simulink model "Machine_Learning"  (R2021b)
settings: Solver=FixedStepAuto  StartTime=0.0  StopTime=1.3  FixedStep=Ts  RelTol=1e-3
model workspace (MAT data in the model file):
  Motor_Gain = 1
values from neighbouring files (symbols this model uses):
  Gain = x(i)    [LS_simulation.m]
  J = 7.65e-3    (= 0.00765)    [Hyperparamter_Optimization.m]    (also in LS_simulation.m)
  Ka = 6.4898    [Hyperparamter_Optimization.m]    (also in LS_simulation.m)
  Kt = 0.4769    [Hyperparamter_Optimization.m]    (also in LS_simulation.m)
  rg = 1.5915    [LS_simulation.m]
settings Model: Creator=user  LastModifiedBy=Duncan
settings SolverCC: AlgebraicLoopSolver=TrustRegion
settings DebuggingCC: SFMachineParentedDataDiag=warning

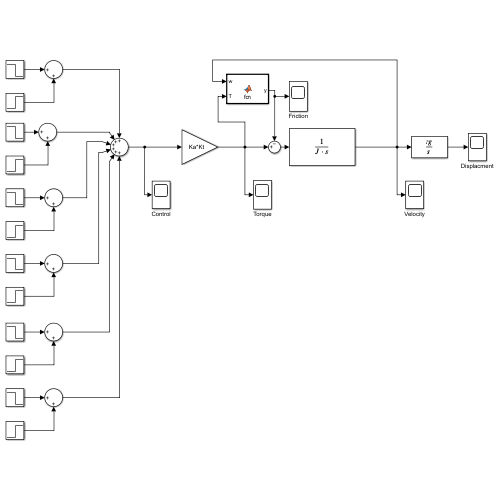
[thumbnail: Simulink's stored preview of the top-level diagram]
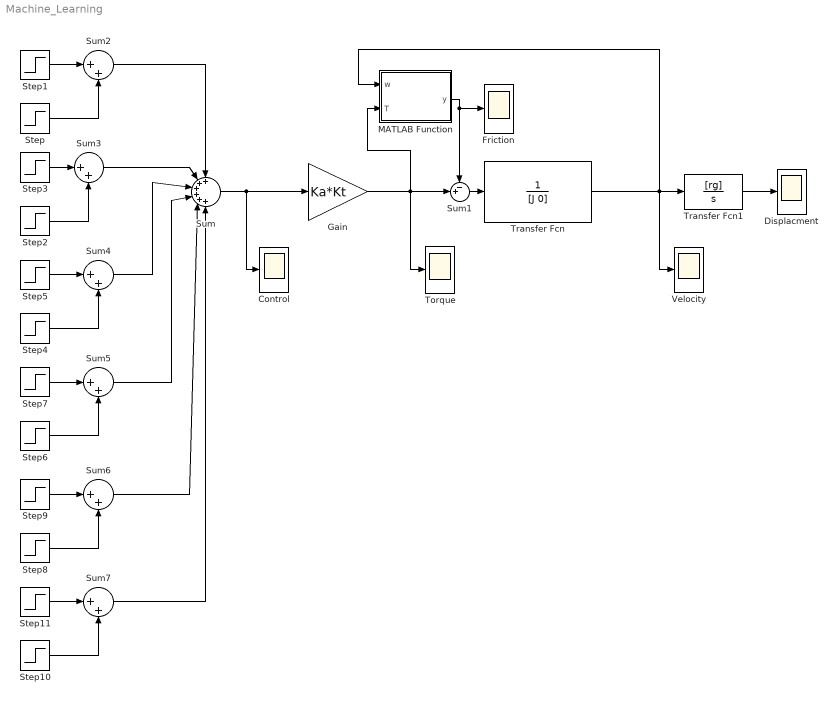
== system Machine_Learning ==
  Control : Scope
  Displacment : Scope
  Friction : Scope
  Gain : Gain  Gain=Ka*Kt
  MATLAB Function : MATLAB Function  TreatAsAtomicUnit=on
  Step : Step  Time=0.2  After=0.2*Gain  SampleTime=0
  Step1 : Step  Time=0.1  After=-0.1*Gain  SampleTime=0
  Step10 : Step  Time=1.2  After=0.1*Gain  SampleTime=0
  Step11 : Step  Time=1.1  After=-0.2*Gain  SampleTime=0
  Step2 : Step  Time=0.4  After=0.4*Gain  SampleTime=0
  Step3 : Step  Time=0.3  After=-0.3*Gain  SampleTime=0
  Step4 : Step  Time=0.6  After=0.6*Gain  SampleTime=0
  Step5 : Step  Time=0.5  After=-0.5*Gain  SampleTime=0
  Step6 : Step  Time=0.8  After=0.5*Gain  SampleTime=0
  Step7 : Step  Time=0.7  After=-0.6*Gain  SampleTime=0
  Step8 : Step  After=0.3*Gain  SampleTime=0
  Step9 : Step  Time=0.9  After=-0.4*Gain  SampleTime=0
  Sum : Sum  Inputs=++++++
  Sum1 : Sum  Inputs=-+|
  Sum{2..7} (6 alike) : Sum  Inputs=|++
  Torque : Scope
  Transfer Fcn : TransferFcn  Denominator=[J 0]
  Transfer Fcn1 : TransferFcn  Numerator=[rg]  Denominator=[1 0]
  Velocity : Scope
  wires:
  Gain/1 -> MATLAB Function/2(T), Sum1/2, Torque/1
  Sum1/1 -> Transfer Fcn/1
  MATLAB Function/1(y) -> Friction/1, Sum1/1
  Transfer Fcn1/1 -> Displacment/1
  Step1/1 -> Sum2/1
  Sum2/1 -> Sum/1
  Sum3/1 -> Sum/2
  Sum4/1 -> Sum/3
  Sum5/1 -> Sum/4
  Sum6/1 -> Sum/5
  Sum7/1 -> Sum/6
  Step/1 -> Sum2/2
  Step3/1 -> Sum3/1
  Step2/1 -> Sum3/2
  Step5/1 -> Sum4/1
  Step4/1 -> Sum4/2
  Step6/1 -> Sum5/2
  Step7/1 -> Sum5/1
  Step9/1 -> Sum6/1
  Step8/1 -> Sum6/2
  Step11/1 -> Sum7/1
  Step10/1 -> Sum7/2
  Transfer Fcn/1 -> MATLAB Function/1(w), Velocity/1, Transfer Fcn1/1
  Sum/1 -> Control/1, Gain/1

== matlab function Machine_Learning/MATLAB Function ==
  data: w input; T input; y output
function y = fcn(w, T)
    %Friction Values
    Tpstat = 3.647;
    Tmstat = -2.702;
    Tpcoul = 2.205;
    Tmcoul = -1.656;
    B = 0.0321;
    Op = 2;
    Om = -2;
    %Friction Function
    if w > 0
        y = Tpstat*exp(-w/Op)+Tpcoul*(1-exp(-w/Op))+B*w;
    elseif w < 0
        y = Tmstat*exp(-w/Om)+Tmcoul*(1-exp(-w/Om))+B*w;
    elseif T>0 && T<Tpstat && w==0
        y = T;
    elseif T<0 && T>Tmstat && w==0
        y = T;
    elseif T>0 && T>Tpstat && w==0
        y = Tpstat;
    elseif T<0 && T<Tmstat && w==0
        y = Tmstat;
    else
        y = 0;
    end
end
